simulink model "Pole_Placement_test"  (R2020a)
settings: Solver=VariableStepAuto  StartTime=0.0  StopTime=40  RelTol=1e-3
values from neighbouring files (symbols this model uses):
  down = -up    (= -0.10471975512)    [Discrete_pole_placement.m]    (also in Pole_Placement_PID.m = -0.0872664625997)
  Kx = place(A_x,1.2*B_x,p)    [Pole_Placement_PID.m]
  Ky = place(A_y,1.2*B_y,p)    [Pole_Placement_PID.m]
  up = 6*pi/180    (= 0.10471975512)    [Discrete_pole_placement.m]    (also in Pole_Placement_PID.m = 0.0872664625997)
settings Model: Creator=Ashraf  LastModifiedBy=hhiastt
settings DataIOCC: ReturnWorkspaceOutputs=off
settings DebuggingCC: ArithmeticOperatorsInVariantConditions=warning
settings SFSimCC: SimUseLocalCustomCode=off  CustomCodeUndefinedFunction=UseInterfaceOnly
settings RTWCC: RTWUseLocalCustomCode=off
settings CodeAppCC: StateflowObjectComments=on

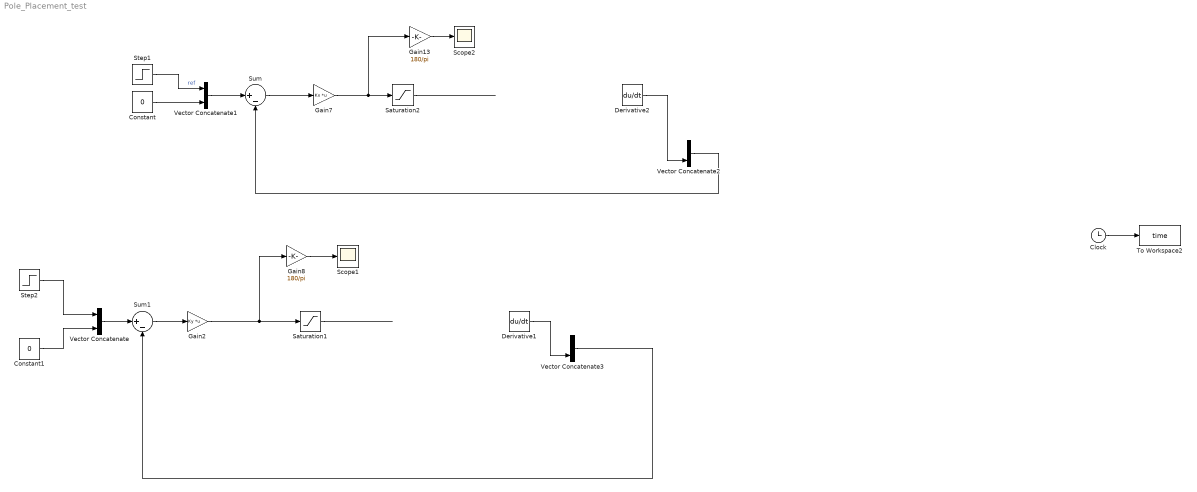
== system Pole_Placement_test ==
  Clock : Clock
  Constant : Constant  Value=0
  Constant1 : Constant  Value=0
  Derivative1 : Derivative
  Derivative2 : Derivative
  Gain13 : Gain  Gain=180/pi
  Gain2 : Gain  Gain=Ky  Multiplication=Matrix(K*u)
  Gain7 : Gain  Gain=Kx  Multiplication=Matrix(K*u)
  Gain8 : Gain  Gain=180/pi
  Saturation1 : Saturate  UpperLimit=up  LowerLimit=down
  Saturation2 : Saturate  UpperLimit=up  LowerLimit=down
  Scope1 : Scope
  Scope2 : Scope
  Step1 : Step  Time=0  After=0.1  SampleTime=0
  Step2 : Step  Time=0  After=0.1  SampleTime=0
  Sum : Sum  Inputs=|+-
  Sum1 : Sum  Inputs=|+-
  To Workspace2 : ToWorkspace  VariableName=time  SampleTime=-1
  Vector Concatenate{,1..3} (4 alike) : Concatenate
  wires:
  Clock/1 -> To Workspace2/1
  Gain13/1 -> Scope2/1
  ? -> Derivative2/1, Vector Concatenate2/1
  Sum/1 -> Gain7/1
  Vector Concatenate3/1 -> Sum1/2
  Gain8/1 -> Scope1/1
  Sum1/1 -> Gain2/1
  Gain7/1 -> Saturation2/1, Gain13/1
  Step2/1 -> Vector Concatenate/1
  Saturation1/1 -> ?
  ? -> Vector Concatenate3/1, Derivative1/1
  Vector Concatenate1/1 -> Sum/1
  Vector Concatenate/1 -> Sum1/1
  Gain2/1 -> Saturation1/1, Gain8/1
  Step1/1 -> Vector Concatenate1/1  "ref"
  Derivative2/1 -> Vector Concatenate2/2
  Vector Concatenate2/1 -> Sum/2
  Constant/1 -> Vector Concatenate1/2
  Constant1/1 -> Vector Concatenate/2
  Saturation2/1 -> ?
  Derivative1/1 -> Vector Concatenate3/2
